simulink model "LR"  (R2024b)
settings: Solver=FixedStepAuto  StartTime=0.0  StopTime=Inf  FixedStep=0.001  RelTol=1e-3
settings Model: Creator=sung  LastModifiedBy=sung
settings HardwareCC: ProdBitPerLong=64  ProdLongLongMode=on  ProdHWDeviceType=Intel->x86-64 (Linux 64)
settings RTWCC: GenCodeOnly=on  Toolchain=CMake

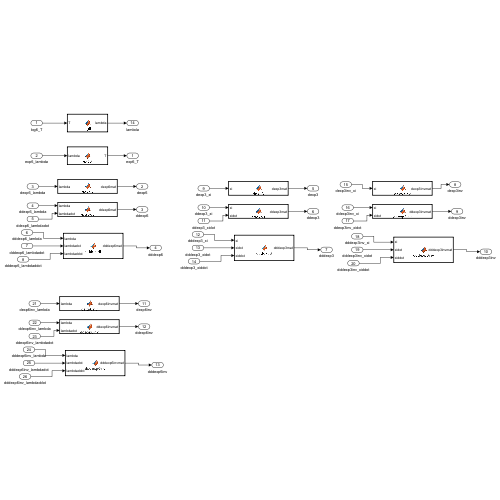
[thumbnail: Simulink's stored preview of the top-level diagram]
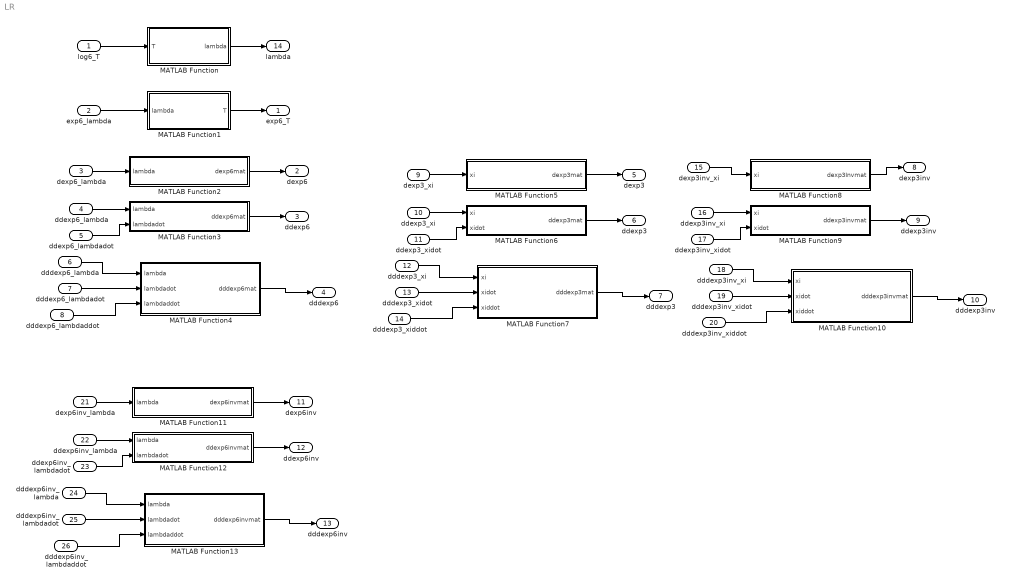
== system LR ==
  log6_T : Inport  PortDimensions=[4,4]
  exp6_lambda : Inport  Port=2  PortDimensions=6
  dexp6_lambda : Inport  Port=3  PortDimensions=6
  ddexp6_lambda : Inport  Port=4  PortDimensions=6
  ddexp6_lambdadot : Inport  Port=5  PortDimensions=6
  dddexp6_lambda : Inport  Port=6  PortDimensions=6
  dddexp6_lambdadot : Inport  Port=7  PortDimensions=6
  dddexp6_lambdaddot : Inport  Port=8  PortDimensions=6
  dexp3_xi : Inport  Port=9  PortDimensions=3
  ddexp3_xi : Inport  Port=10  PortDimensions=3
  ddexp3_xidot : Inport  Port=11  PortDimensions=3
  dddexp3_xi : Inport  Port=12  PortDimensions=3
  dddexp3_xidot : Inport  Port=13  PortDimensions=3
  dddexp3_xiddot : Inport  Port=14  PortDimensions=3
  dexp3inv_xi : Inport  Port=15  PortDimensions=6
  ddexp3inv_xi : Inport  Port=16  PortDimensions=3
  ddexp3inv_xidot : Inport  Port=17  PortDimensions=3
  dddexp3inv_xi : Inport  Port=18  PortDimensions=3
  dddexp3inv_xidot : Inport  Port=19  PortDimensions=3
  dddexp3inv_xiddot : Inport  Port=20  PortDimensions=3
  dexp6inv_lambda : Inport  Port=21  PortDimensions=6
  ddexp6inv_lambda : Inport  Port=22  PortDimensions=6
  ddexp6inv_lambdadot : Inport  Port=23  PortDimensions=6
  dddexp6inv_lambda : Inport  Port=24  PortDimensions=6
  dddexp6inv_lambdadot : Inport  Port=25  PortDimensions=6
  dddexp6inv_lambdaddot : Inport  Port=26  PortDimensions=6
  MATLAB Function : MATLAB Function  TreatAsAtomicUnit=on
  MATLAB Function1 : MATLAB Function  TreatAsAtomicUnit=on
  MATLAB Function10 : MATLAB Function  TreatAsAtomicUnit=on
  MATLAB Function11 : MATLAB Function  TreatAsAtomicUnit=on
  MATLAB Function12 : MATLAB Function  TreatAsAtomicUnit=on
  MATLAB Function13 : MATLAB Function  TreatAsAtomicUnit=on
  MATLAB Function2 : MATLAB Function  TreatAsAtomicUnit=on
  MATLAB Function3 : MATLAB Function  TreatAsAtomicUnit=on
  MATLAB Function4 : MATLAB Function  TreatAsAtomicUnit=on
  MATLAB Function5 : MATLAB Function  TreatAsAtomicUnit=on
  MATLAB Function6 : MATLAB Function  TreatAsAtomicUnit=on
  MATLAB Function7 : MATLAB Function  TreatAsAtomicUnit=on
  MATLAB Function8 : MATLAB Function  TreatAsAtomicUnit=on
  MATLAB Function9 : MATLAB Function  TreatAsAtomicUnit=on
  exp6_T : Outport  PortDimensions=[4,4]
  dexp6 : Outport  Port=2  PortDimensions=[6,6]
  ddexp6 : Outport  Port=3  PortDimensions=[6,6]
  dddexp6 : Outport  Port=4  PortDimensions=[6,6]
  dexp3 : Outport  Port=5  PortDimensions=[3,3]
  ddexp3 : Outport  Port=6  PortDimensions=[3,3]
  dddexp3 : Outport  Port=7  PortDimensions=[3,3]
  dexp3inv : Outport  Port=8  PortDimensions=[3,3]
  ddexp3inv : Outport  Port=9  PortDimensions=[3,3]
  dddexp3inv : Outport  Port=10  PortDimensions=[3,3]
  dexp6inv : Outport  Port=11  PortDimensions=[6,6]
  ddexp6inv : Outport  Port=12  PortDimensions=[6,6]
  dddexp6inv : Outport  Port=13  PortDimensions=[6,6]
  lambda : Outport  Port=14  PortDimensions=6
  wires:
  log6_T/1 -> MATLAB Function/1(T)
  MATLAB Function1/1(T) -> exp6_T/1
  exp6_lambda/1 -> MATLAB Function1/1(lambda)
  dexp6_lambda/1 -> MATLAB Function2/1(lambda)
  MATLAB Function2/1(dexp6mat) -> dexp6/1
  ddexp6_lambda/1 -> MATLAB Function3/1(lambda)
  MATLAB Function3/1(ddexp6mat) -> ddexp6/1
  ddexp6_lambdadot/1 -> MATLAB Function3/2(lambdadot)
  dddexp6_lambda/1 -> MATLAB Function4/1(lambda)
  dddexp6_lambdadot/1 -> MATLAB Function4/2(lambdadot)
  dddexp6_lambdaddot/1 -> MATLAB Function4/3(lambdaddot)
  MATLAB Function4/1(dddexp6mat) -> dddexp6/1
  MATLAB Function6/1(ddexp3mat) -> ddexp3/1
  ddexp3_xi/1 -> MATLAB Function6/1(xi)
  dddexp3_xidot/1 -> MATLAB Function7/2(xidot)
  dddexp3_xiddot/1 -> MATLAB Function7/3(xiddot)
  dexp3_xi/1 -> MATLAB Function5/1(xi)
  dddexp3_xi/1 -> MATLAB Function7/1(xi)
  ddexp3_xidot/1 -> MATLAB Function6/2(xidot)
  MATLAB Function7/1(dddexp3mat) -> dddexp3/1
  MATLAB Function5/1(dexp3mat) -> dexp3/1
  MATLAB Function8/1(dexp3Invmat) -> dexp3inv/1
  dexp3inv_xi/1 -> MATLAB Function8/1(xi)
  ddexp3inv_xi/1 -> MATLAB Function9/1(xi)
  ddexp3inv_xidot/1 -> MATLAB Function9/2(xidot)
  MATLAB Function9/1(ddexp3invmat) -> ddexp3inv/1
  dddexp3inv_xiddot/1 -> MATLAB Function10/3(xiddot)
  dddexp3inv_xi/1 -> MATLAB Function10/1(xi)
  dddexp3inv_xidot/1 -> MATLAB Function10/2(xidot)
  MATLAB Function10/1(dddexp3invmat) -> dddexp3inv/1
  MATLAB Function12/1(ddexp6invmat) -> ddexp6inv/1
  ddexp6inv_lambda/1 -> MATLAB Function12/1(lambda)
  dddexp6inv_lambdadot/1 -> MATLAB Function13/2(lambdadot)
  dddexp6inv_lambdaddot/1 -> MATLAB Function13/3(lambdaddot)
  dexp6inv_lambda/1 -> MATLAB Function11/1(lambda)
  dddexp6inv_lambda/1 -> MATLAB Function13/1(lambda)
  ddexp6inv_lambdadot/1 -> MATLAB Function12/2(lambdadot)
  MATLAB Function13/1(dddexp6invmat) -> dddexp6inv/1
  MATLAB Function11/1(dexp6invmat) -> dexp6inv/1
  MATLAB Function/1(lambda) -> lambda/1

== matlab function LR/MATLAB Function12 ==
  data: lambda input; ddexp6invmat output; lambdadot input
function ddexp6invmat = ddexp6inv(lambda,lambdadot)

ddexp6invmat = ddlog6(lambda,lambdadot);

== matlab function LR/MATLAB Function13 ==
  data: lambda input; dddexp6invmat output; lambdadot input; lambdaddot input
function dddexp6invmat = dddexp6inv(lambda,lambdadot,lambdaddot)

dddexp6invmat = dddlog6(lambda,lambdadot,lambdaddot);

== matlab function LR/MATLAB Function ==
  data: T input; lambda output
function lambda = log6(T)
if(norm(T) <eps) T= eye(4);
end
lambda = log6(T);

== matlab function LR/MATLAB Function2 ==
  data: lambda input; dexp6mat output
function dexp6mat = dexp6(lambda)

dexp6mat = dexp6(lambda);

== matlab function LR/MATLAB Function3 ==
  data: lambda input; ddexp6mat output; lambdadot input
function ddexp6mat = ddexp6(lambda,lambdadot)

ddexp6mat = ddexp6(lambda,lambdadot);

== matlab function LR/MATLAB Function4 ==
  data: lambda input; dddexp6mat output; lambdadot input; lambdaddot input
function dddexp6mat = dddexp6(lambda,lambdadot,lambdaddot)

dddexp6mat = dddexp6(lambda,lambdadot,lambdaddot);

== matlab function LR/MATLAB Function5 ==
  data: xi input; dexp3mat output
function dexp3mat = dexp3(xi)

dexp3mat = dexp3(xi);

== matlab function LR/MATLAB Function6 ==
  data: xi input; ddexp3mat output; xidot input
function ddexp3mat = ddexp3(xi,xidot)

ddexp3mat = ddexp3(xi,xidot);

== matlab function LR/MATLAB Function7 ==
  data: xi input; dddexp3mat output; xidot input; xiddot input
function dddexp3mat = dddexp3(xi,xidot,xiddot)

dddexp3mat = dddexp3(xi,xidot,xiddot);

== matlab function LR/MATLAB Function8 ==
  data: xi input; dexp3Invmat output
function dexp3Invmat = dexp3Inv(xi)

dexp3Invmat = dlog3(xi);

== matlab function LR/MATLAB Function9 ==
  data: xi input; ddexp3invmat output; xidot input
function ddexp3invmat = ddexp3inv(xi,xidot)

ddexp3invmat = ddlog3(xi,xidot);

== matlab function LR/MATLAB Function10 ==
  data: xi input; dddexp3invmat output; xidot input; xiddot input
function dddexp3invmat = dddexp3inv(xi,xidot,xiddot)

dddexp3invmat = dddlog3(xi,xidot,xiddot);

== matlab function LR/MATLAB Function1 ==
  data: lambda input; T output
function T = exp6(lambda)

T = exp6(lambda);

== matlab function LR/MATLAB Function11 ==
  data: lambda input; dexp6invmat output
function dexp6invmat = dexp6inv(lambda)

dexp6invmat = dlog6(lambda);
